simulink library "SEIR_Lib"  (R2019b)
settings: Solver=VariableStepAuto  StartTime=0.0  StopTime=10.0  RelTol=1e-3
undefined symbols (not defined in the file or in its folder): sigbuilder_block
libraries: $bdroot x4
settings Model: Creator=Alex  LastModifiedBy=Alex

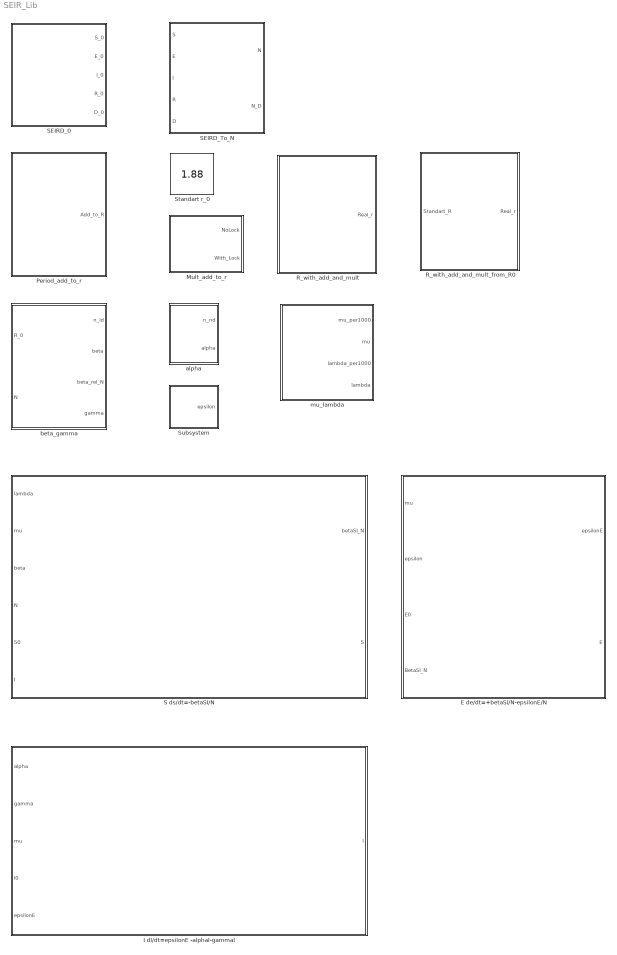
== system SEIR_Lib ==
  E de/dt=+betaSI/N-epsilonE/N : Subsystem
  I dI/dt=epsilonE -alphaI-gammaI : Subsystem
  Mult_add_to_r : Subsystem
  Period_add_to_r : Subsystem
  R_with_add_and_mult : Subsystem
  R_with_add_and_mult_from_R0 : Subsystem
  S ds/dt=-betaSI/N : Subsystem
  SEIRD_0 : Subsystem
  SEIRD_To_N : Subsystem
  Standart r_0 : Constant  Value=1.88
  Subsystem : Subsystem
  alpha : Subsystem
  beta_gamma : Subsystem
  mu_lambda : Subsystem

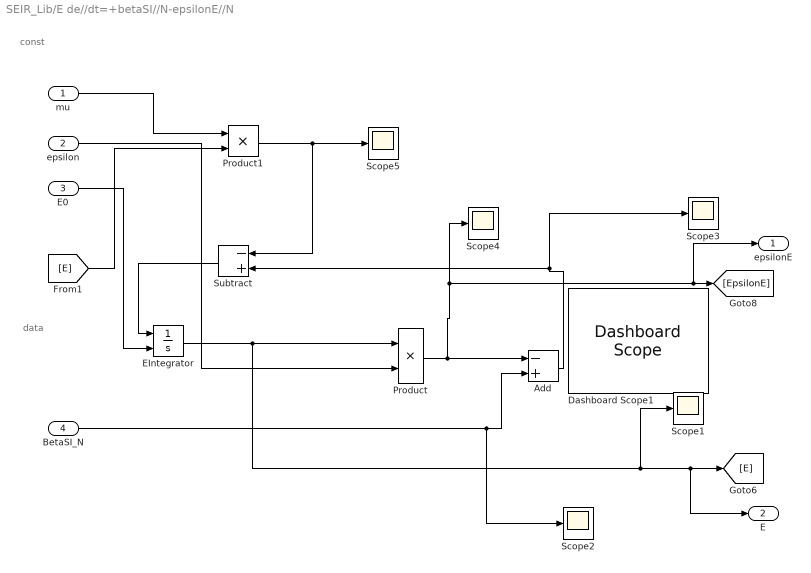
== system SEIR_Lib/E de//dt=+betaSI//N-epsilonE//N ==
  note: data
  note: const
  mu : Inport
  epsilon : Inport  Port=2
  E0 : Inport  Port=3
  BetaSI_N : Inport  Port=4
  Add : Sum  Inputs=-+
  Dashboard Scope1 : DashboardScope
  EIntegrator : Integrator  InitialConditionSource=external
  Product : Product  Inputs=**
  Product1 : Product
  Scope{1..5} (5 alike) : Scope
  Subtract : Sum  Inputs=-+
  epsilonE : Outport
  E : Outport  Port=2
  wires:
  E0/1 -> EIntegrator/2
  Product1/1 -> Scope5/1, Subtract/1
  BetaSI_N/1 -> Scope2/1, Add/2
  Add/1 -> Subtract/2, Scope3/1
  mu/1 -> Product1/1
  epsilon/1 -> Product/2
  Product/1 -> Scope4/1, epsilonE/1, [EpsilonE], Add/1
  EIntegrator/1 -> Scope1/1, E/1, [E], Product/1
  [E] -> Product1/2
  Subtract/1 -> EIntegrator/1

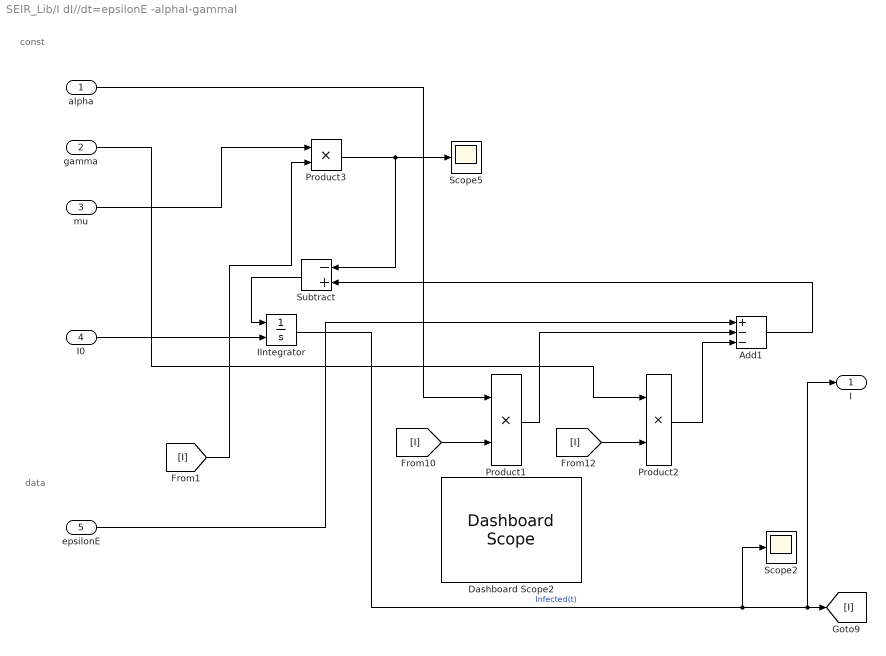
== system SEIR_Lib/I dI//dt=epsilonE -alphaI-gammaI ==
  note: data
  note: const
  alpha : Inport
  gamma : Inport  Port=2
  mu : Inport  Port=3
  I0 : Inport  Port=4
  epsilonE : Inport  Port=5
  Add1 : Sum  Inputs=+--
  Dashboard Scope2 : DashboardScope  Ymax=150e6
  IIntegrator : Integrator  InitialConditionSource=external
  Product1 : Product  Inputs=**
  Product2 : Product  Inputs=**
  Product3 : Product
  Scope2 : Scope
  Scope5 : Scope
  Subtract : Sum  Inputs=-+
  I : Outport
  wires:
  Add1/1 -> Subtract/2
  IIntegrator/1 -> I/1, [I], Scope2/1  "Infected(t)"
  I0/1 -> IIntegrator/2
  [I] -> Product1/2
  Subtract/1 -> IIntegrator/1
  gamma/1 -> Product2/1
  Product1/1 -> Add1/2
  Product2/1 -> Add1/3
  mu/1 -> Product3/1
  [I] -> Product3/2
  Product3/1 -> Scope5/1, Subtract/1
  [I] -> Product2/2
  alpha/1 -> Product1/1
  epsilonE/1 -> Add1/1

== system SEIR_Lib/Mult_add_to_r ==
  note: s2 = 1
      | s1 = 1 0. 5 0.8...
  Signal Builder : Subsystem  Tag=STV Subsys  LoadFcn=sigbuilder_block('load');  StartFcn=sigbuilder_block('start');  StopFcn=sigbuilder_block('stop');  ClipboardFcn=sigbuilder_block('clipboard');  mask(Sigbuilder block){tuvar=[0:10]}
      mask help: Simulink:masks:SigbuilderBlock_MD
      mask init:
      | if ~strcmp(get_param(bdroot(gcbh),'SimulationStatus'),'stopped') tuvar = sigbuilder_block('maskInit'); end
      settings: CopyFcn=sigbuilder_block('copy');  DeleteFcn=sigbuilder_block('delete');  ModelCloseFcn=sigbuilder_block('modelClose');  PreSaveFcn=sigbuilder_block('preSave');  PauseFcn=sigbuilder_block('pause');  ContinueFcn=sigbuilder_block('continue');  NameChangeFcn=sigbuilder_block('namechange');  OpenFcn=sigbuilder_block('open',[437.6 199.2 550.4 400 ]);  CloseFcn=sigbuilder_block('close');
      mask Display: plot(0, 0, 100, 100,[2, 2, 32, 32, 2], [68, 8, 8, 68, 68],[32, 2], [38, 38], [32, 19, 2],[53, 60, 44], [32, 17, 17, 2],[16, 16, 31, 31]);txt = getActiveGroup(gcbh);text(2, 100, txt,'verticalAlignment', 'top');
  NoLock : Outport
  With_Lock : Outport  Port=2
  wires:
  Signal Builder/1(Signal 2) -> NoLock/1
  Signal Builder/2(Signal 1) -> With_Lock/1

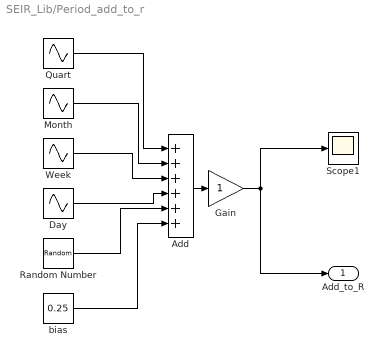
== system SEIR_Lib/Period_add_to_r ==
  Add : Sum  Inputs=++++++
  Day : Sin  Amplitude=0.12*2  Frequency=2*pi/7  SampleTime=0
  Gain : Gain
  Month : Sin  Amplitude=0.12  Frequency=2*pi/30  SampleTime=0
  Quart : Sin  Amplitude=0.12  Frequency=2*pi/120  SampleTime=0
  Random Number : RandomNumber  Variance=0.0144  SampleTime=0.1
  Scope1 : Scope
  Week : Sin  Amplitude=0.12  Frequency=2*pi/7  SampleTime=0
  bias : Constant  Value=0.25
  Add_to_R : Outport
  wires:
  Gain/1 -> Add_to_R/1, Scope1/1
  Month/1 -> Add/2
  Week/1 -> Add/3
  bias/1 -> Add/6
  Quart/1 -> Add/1
  Random Number/1 -> Add/5
  Add/1 -> Gain/1
  Day/1 -> Add/4

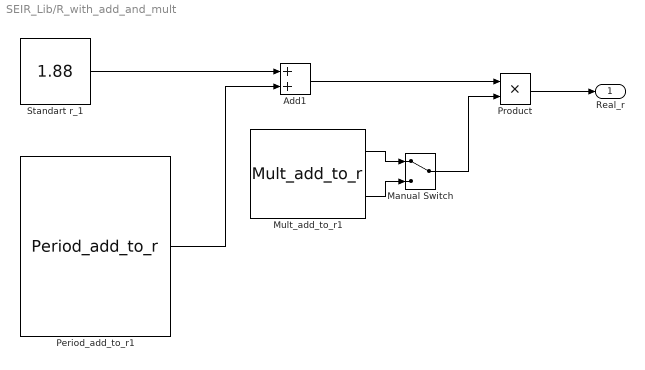
== system SEIR_Lib/R_with_add_and_mult ==
  Add1 : Sum
  Manual Switch : ManualSwitch
  Mult_add_to_r1 : $bdroot/Mult_add_to_r  SystemSampleTime=-1  Latency=0  AutoFrameSizeCalculation=off
  Period_add_to_r1 : $bdroot/Period_add_to_r  SystemSampleTime=-1  Latency=0  AutoFrameSizeCalculation=off
  Product : Product
  Standart r_1 : Constant  Value=1.88
  Real_r : Outport
  wires:
  Period_add_to_r1/1 -> Add1/2
  Standart r_1/1 -> Add1/1
  Manual Switch/1 -> Product/2
  Add1/1 -> Product/1
  Mult_add_to_r1/1 -> Manual Switch/1
  Mult_add_to_r1/2 -> Manual Switch/2
  Product/1 -> Real_r/1

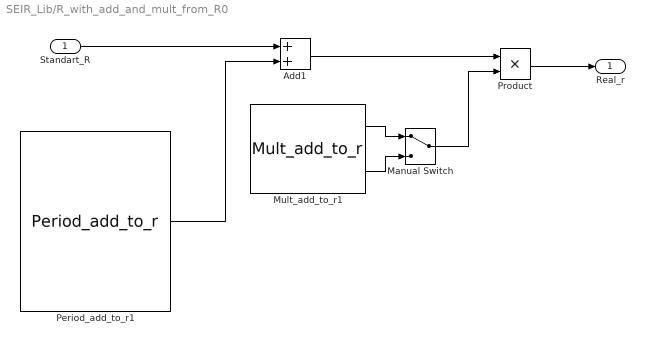
== system SEIR_Lib/R_with_add_and_mult_from_R0 ==
  Standart_R : Inport
  Add1 : Sum
  Manual Switch : ManualSwitch
  Mult_add_to_r1 : $bdroot/Mult_add_to_r  SystemSampleTime=-1  Latency=0  AutoFrameSizeCalculation=off
  Period_add_to_r1 : $bdroot/Period_add_to_r  SystemSampleTime=-1  Latency=0  AutoFrameSizeCalculation=off
  Product : Product
  Real_r : Outport
  wires:
  Product/1 -> Real_r/1
  Mult_add_to_r1/2 -> Manual Switch/2
  Mult_add_to_r1/1 -> Manual Switch/1
  Add1/1 -> Product/1
  Manual Switch/1 -> Product/2
  Standart_R/1 -> Add1/1
  Period_add_to_r1/1 -> Add1/2

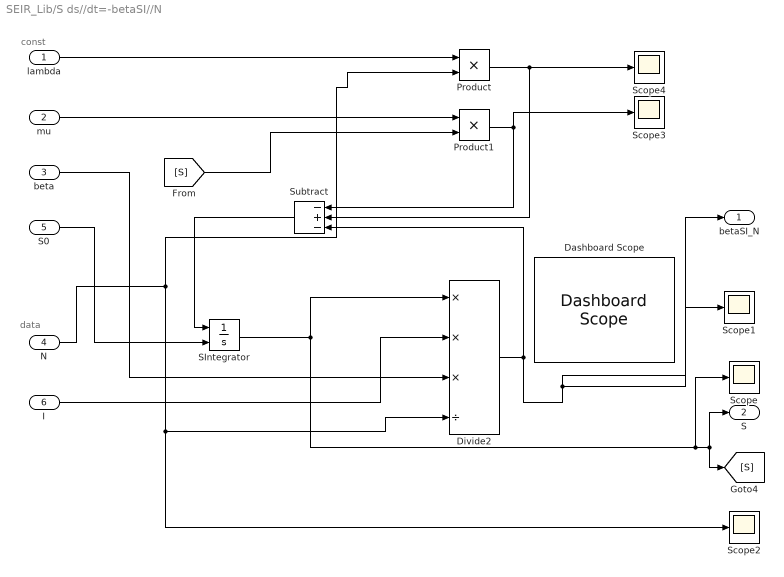
== system SEIR_Lib/S ds//dt=-betaSI//N ==
  note: data
  note: const
  lambda : Inport
  mu : Inport  Port=2
  beta : Inport  Port=3
  N : Inport  Port=4
  S0 : Inport  Port=5
  I : Inport  Port=6
  Dashboard Scope : DashboardScope  Ymax=150e6
  Divide2 : Product  Inputs=***/
  Product : Product
  Product1 : Product
  SIntegrator : Integrator  InitialConditionSource=external
  Scope{,1..4} (5 alike) : Scope
  Subtract : Sum  Inputs=-+-
  betaSI_N : Outport
  S : Outport  Port=2
  wires:
  Divide2/1 -> Subtract/3, betaSI_N/1, Scope1/1
  SIntegrator/1 -> Scope/1, S/1, [S], Divide2/1
  N/1 -> Product/2, Scope2/1, Divide2/4
  beta/1 -> Divide2/3
  I/1 -> Divide2/2
  S0/1 -> SIntegrator/2
  Subtract/1 -> SIntegrator/1
  mu/1 -> Product1/1
  [S] -> Product1/2
  Product1/1 -> Subtract/1, Scope3/1
  lambda/1 -> Product/1
  Product/1 -> Scope4/1, Subtract/2

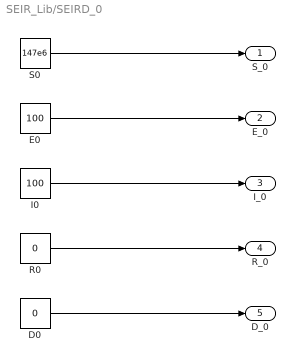
== system SEIR_Lib/SEIRD_0 ==
  D0 : Constant  Value=0
  E0 : Constant  Value=100
  I0 : Constant  Value=100
  R0 : Constant  Value=0
  S0 : Constant  Value=147e6
  S_0 : Outport
  E_0 : Outport  Port=2
  I_0 : Outport  Port=3
  R_0 : Outport  Port=4
  D_0 : Outport  Port=5
  wires:
  D0/1 -> D_0/1
  S0/1 -> S_0/1
  I0/1 -> I_0/1
  E0/1 -> E_0/1
  R0/1 -> R_0/1

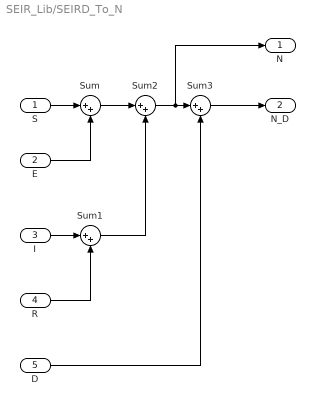
== system SEIR_Lib/SEIRD_To_N ==
  S : Inport
  E : Inport  Port=2
  I : Inport  Port=3
  R : Inport  Port=4
  D : Inport  Port=5
  Sum{,1..3} (4 alike) : Sum  Inputs=|++
  N : Outport
  N_D : Outport  Port=2
  wires:
  Sum1/1 -> Sum2/2
  S/1 -> Sum/1
  Sum/1 -> Sum2/1
  E/1 -> Sum/2
  I/1 -> Sum1/1
  R/1 -> Sum1/2
  Sum2/1 -> N/1, Sum3/1
  Sum3/1 -> N_D/1
  D/1 -> Sum3/2

== system SEIR_Lib/Subsystem ==
  Product4 : Product
  Random NumberEpsilon : RandomNumber  Mean=1  SampleTime=0.1
  Scope6 : Scope
  epsilon_const : Constant  Value=3.33
  epsilon : Outport
  wires:
  Random NumberEpsilon/1 -> Product4/2
  Product4/1 -> Scope6/1, epsilon/1, [epsilon]
  epsilon_const/1 -> Product4/1

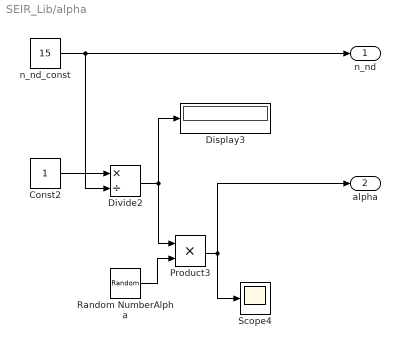
== system SEIR_Lib/alpha ==
  Const2 : Constant
  Display3 : Display
  Divide2 : Product  Inputs=*/
  Product3 : Product
  Random NumberAlpha : RandomNumber  Mean=1  Variance=50e-6  SampleTime=0.1
  Scope4 : Scope
  n_nd_const : Constant  Value=15
  n_nd : Outport
  alpha : Outport  Port=2
  wires:
  Random NumberAlpha/1 -> Product3/2
  Divide2/1 -> Product3/1, Display3/1
  n_nd_const/1 -> n_nd/1, Divide2/2
  Product3/1 -> alpha/1, Scope4/1
  Const2/1 -> Divide2/1

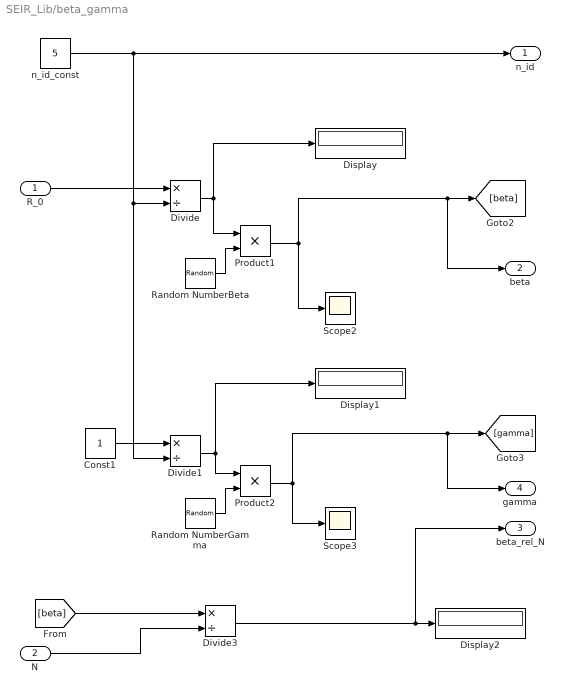
== system SEIR_Lib/beta_gamma ==
  R_0 : Inport
  N : Inport  Port=2
  Const1 : Constant
  Display : Display
  Display1 : Display
  Display2 : Display
  Divide : Product  Inputs=*/
  Divide1 : Product  Inputs=*/
  Divide3 : Product  Inputs=*/
  Product1 : Product
  Product2 : Product
  Random NumberBeta : RandomNumber  Mean=1  Variance=0.0016  SampleTime=0.1
  Random NumberGamma : RandomNumber  Mean=1  Variance=0.0008  SampleTime=0.1
  Scope2 : Scope
  Scope3 : Scope
  n_id_const : Constant  Value=5
  n_id : Outport
  beta : Outport  Port=2
  beta_rel_N : Outport  Port=3
  gamma : Outport  Port=4
  wires:
  R_0/1 -> Divide/1
  Random NumberGamma/1 -> Product2/2
  Product2/1 -> Scope3/1, gamma/1, [gamma]
  Divide1/1 -> Product2/1, Display1/1
  Product1/1 -> Scope2/1, beta/1, [beta]
  Divide3/1 -> beta_rel_N/1, Display2/1
  [beta] -> Divide3/1
  Random NumberBeta/1 -> Product1/2
  Const1/1 -> Divide1/1
  n_id_const/1 -> n_id/1, Divide1/2, Divide/2
  Divide/1 -> Product1/1, Display/1
  N/1 -> Divide3/2

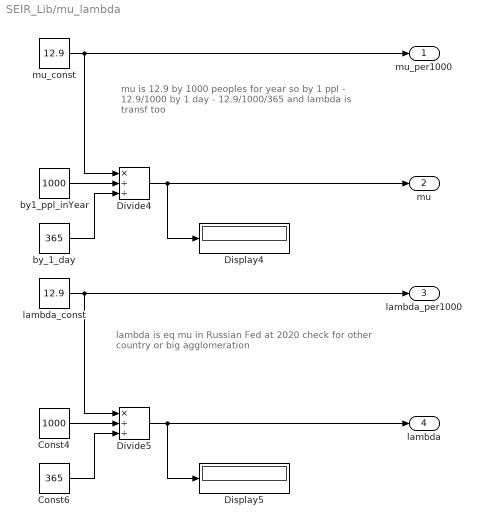
== system SEIR_Lib/mu_lambda ==
  note: mu is 12.9 by 1000 peoples for year
      | so by 1 ppl - 12.9/1000
      | by 1 day - 12.9/1000/365
      | and lambda is transf too
  note: lambda is eq mu in Russian Fed at 2020
      | check for other country or big agglomeration
  Const4 : Constant  Value=1000
  Const6 : Constant  Value=365
  Display4 : Display
  Display5 : Display
  Divide4 : Product  Inputs=*//
  Divide5 : Product  Inputs=*//
  by1_ppl_inYear : Constant  Value=1000
  by_1_day : Constant  Value=365
  lambda_const : Constant  Value=12.9
  mu_const : Constant  Value=12.9
  mu_per1000 : Outport
  mu : Outport  Port=2
  lambda_per1000 : Outport  Port=3
  lambda : Outport  Port=4
  wires:
  mu_const/1 -> mu_per1000/1, Divide4/1
  by1_ppl_inYear/1 -> Divide4/2
  lambda_const/1 -> lambda_per1000/1, Divide5/1
  Divide4/1 -> mu/1, Display4/1
  by_1_day/1 -> Divide4/3
  Divide5/1 -> lambda/1, Display5/1
  Const6/1 -> Divide5/3
  Const4/1 -> Divide5/2

== system SEIR_Lib/Mult_add_to_r/Signal Builder ==
  Demux : Demux  Tag=STV Demux  Outputs=2
  FromWs : FromWorkspace  Tag=STV FromWs  VariableName=tuvar  SampleTime=0
      SigBuilderData=|
      | common.afterFinalStr = 'Extrapolate'
      | common.sampleTime = 0
      | dataSet.timeRange = [0 365]
      | dataSet.name = 'Group 1'
      | sbobj.Groups.Name = 'Group 1'
      | sbobj.Groups.Signals(1).Name = 'Signal 2'
      | sbobj.Groups.Signals(1).XData = [0 365]
      | sbobj.Groups.Signals(1).YData = [1 1]
      | sbobj.Groups.Signals(2).Name = 'Signal 1'
      | sbobj.Groups.Signals(2).XData = [0 80 85 125 126 186 187 365]
      | sbobj.Groups.Signals(2).YData = [1 1 0.5 0.5 0.8 0.8 0.85 0.85]
      | sbobj.Groups.TimeRange = [0 365]
  Signal 2 : Outport  Tag=STV Outport
  Signal 1 : Outport  Tag=STV Outport  Port=2
  wires:
  FromWs/1 -> Demux/1
  Demux/1 -> Signal 2/1
  Demux/2 -> Signal 1/1
